simulink model "c09f12_01"  (R2012b)
settings: Solver=ode45  StartTime=0.0  StopTime="(2^(7+2))  * (2^8)"  RelTol=1e-3
undefined symbols (not defined in the file): Down, pfb_coeff_gen_calc, Up, xlipgetpartsetting
libraries: xbsIndex_r4 x7044, casper_library_misc x193, xps_library x58, casper_library_delays x50, simulink x16, dspsigops x12, casper_library_flow_control x5, xbsReplacements_r4 x4, casper_library_ffts_twiddle x2, casper_library_multipliers x2, casper_library_reorder x1
(part 6 of 77)

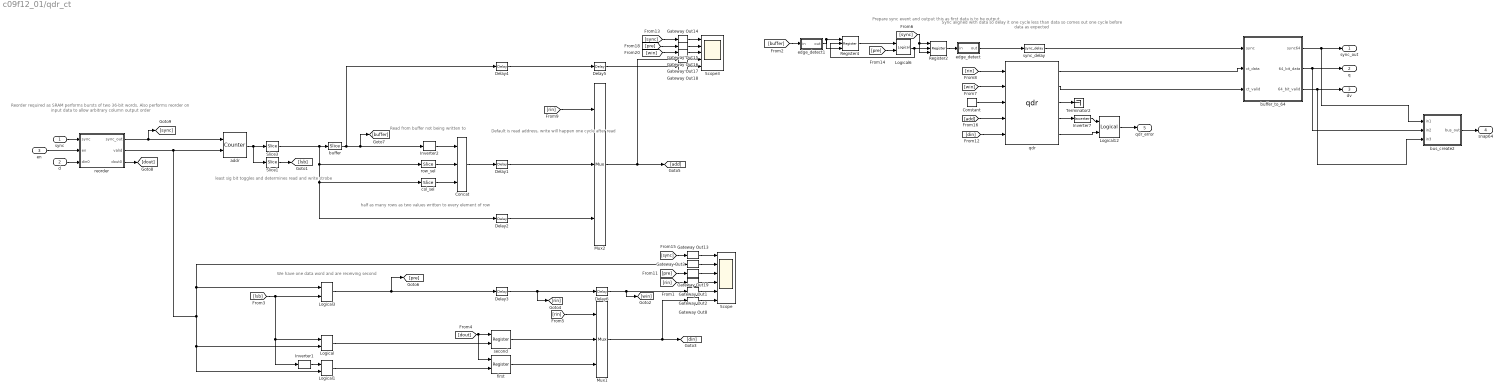
== system c09f12_01/qdr_ct ==
  note: Reorder required as SRAM performs
      | bursts of two 36-bit words.
      | Also performs reorder on input
      | data to allow arbitrary column
      | output order
  note: Prepare sync event and output
      | this as first data is to be output.
  note: Sync aligned with data so
      | delay it one cycle less
      | than data so comes out one
      | cycle before data as
      | expected
  note: least sig bit toggles
      | and determines read
      | and write strobe
  note: We have one data word
      | and are receiving second
  note: Default is read address,
      | write will happen one
      | cycle after read
  note: Read from buffer
      | not being
      | written to
  note: half as many rows
      | as two values
      | written to every
      | element of row
  sync : Inport
  d : Inport  Port=2
  en : Inport  Port=3
  Concat : xbsIndex_r4/Concat  num_inputs=3  dbl_ovrd=off  block_type=concat
      settings: block_version=10.1.3
  Constant : xbsIndex_r4/Constant  const=15  gui_display_data_type=Fixed-point  arith_type=Unsigned  n_bits=4  bin_pt=0  preci_type=Single  exp_width=8  frac_width=24  explicit_period=on  period=1  equ=P=C  opselect=C  inp2=PCIN>>17  opr=+  inp1=P  carry=CIN  dbl_ovrd=off  block_type=constant
  Delay{1..6} (6 alike) : xbsIndex_r4/Delay  rst=off  infoeditControl=Selection of Reset will increase slice count due to use of real FFs and instead of SRLs  en=off  latency=1  dbl_ovrd=off  reg_retiming=off  block_type=delay
      settings: block_version=11.4
  Gateway Out{1..3,8,13..19} (11 alike) : xbsIndex_r4/Gateway Out  inherit_from_input=off  hdl_port=off  timing_constraint=None  locs_specified=off  LOCs={}  UseAsDAC=off  DACChannel='1'  block_type=gatewayout
      settings: infoedit="Gateway out block.  Converts Xilinx fixed point inputs into ouputs of type Simulink integer, double, or fixed point.<br><br>Hardware notes:  In hardware these blocks become top level output ports or are discarded, depending on how they are configured."  block_version=11.4
  Inverter1 : xbsIndex_r4/Inverter  en=off  latency=0  dbl_ovrd=off  block_type=inv
  Inverter2 : xbsIndex_r4/Inverter  en=off  latency=0  dbl_ovrd=off  block_type=inv
  Inverter7 : xbsIndex_r4/Inverter  en=off  latency=0  dbl_ovrd=off  block_type=inv
      settings: block_version=11.4
  Logical{,1,3,6} (4 alike) : xbsIndex_r4/Logical  logical_function=AND  inputs=2  en=off  latency=0  precision=Full  arith_type=Unsigned  n_bits=16  bin_pt=0  align_bp=on  dbl_ovrd=off  block_type=logical
      settings: block_version=11.4
  Logical12 : xbsIndex_r4/Logical  logical_function=OR  inputs=2  en=off  latency=1  precision=Full  arith_type=Unsigned  n_bits=8  bin_pt=2  align_bp=on  dbl_ovrd=off  block_type=logical
      settings: xl_area=[0, 0, 0, 0, 0, 0, 0]
  Mux1 : xbsIndex_r4/Mux  inputs=2  en=off  latency=1  precision=Full  arith_type=Unsigned  n_bits=16  bin_pt=14  quantization=Truncate  overflow=Wrap  dbl_ovrd=off  block_type=mux
      settings: block_version=11.4
  Mux2 : xbsIndex_r4/Mux  inputs=2  en=off  latency=1  precision=Full  arith_type=Unsigned  n_bits=16  bin_pt=14  quantization=Truncate  overflow=Wrap  dbl_ovrd=off  block_type=mux
      settings: block_version=11.4
  Register2 : xbsIndex_r4/Register  init=0  rst=on  en=on  dbl_ovrd=off  block_type=register
      settings: block_version=11.4
  Register4 : xbsIndex_r4/Register  init=0  rst=on  en=on  dbl_ovrd=off  block_type=register
      settings: block_version=11.4
  Scope : Scope  NumInputPorts=6
      settings: YMin=0~0~0~0~0~0  YMax=1~1~1~1~1~15
  Scope3 : Scope  NumInputPorts=5
      settings: TimeRange=27.56125882301808  YMin=0~0~0~0~0  YMax=1~1~600~15~1  SaveName=ScopeData4
  Slice1 : xbsIndex_r4/Slice  nbits=1  boolean_output=on  mode=Lower Bit Location + Width  bit1=0  base1=MSB of Input  bit0=0  base0=LSB of Input  dbl_ovrd=off  block_type=slice
      settings: block_version=10.1.3
  Slice3 : xbsIndex_r4/Slice  nbits=(idepth + odepth + 1) - 1  boolean_output=off  mode=Upper Bit Location + Width  bit1=0  base1=MSB of Input  bit0=0  base0=LSB of Input  dbl_ovrd=off  block_type=slice
      settings: block_version=10.1.3
  Terminator2 : Terminator
  addr : xbsIndex_r4/Counter  cnt_type=Free Running  cnt_to=Inf  operation=Up  start_count=0  cnt_by_val=1  arith_type=Unsigned  n_bits=(idepth + odepth + 1)  bin_pt=0  load_pin=off  rst=on  en=on  explicit_period=on  period=1  dbl_ovrd=off  use_behavioral_HDL=off  implementation=Fabric  use_rpm=off  block_type=counter
  buffer : xbsIndex_r4/Slice  nbits=1  boolean_output=on  mode=Upper Bit Location + Width  bit1=0  base1=MSB of Input  bit0=0  base0=LSB of Input  dbl_ovrd=off  block_type=slice
      settings: block_version=10.1.3
  buffer_to_64 : Subsystem
  bus_create2 : Subsystem  AncestorBlock=casper_library_flow_control/bus_create  mask(bus_create){inputNum=3}
      mask prompts: inputNum "Number of inputs:"
      mask init:
      | bus_create_init(gcb,...
      |     'inputNum', inputNum);
  col_sel : xbsIndex_r4/Slice  nbits=idepth  boolean_output=off  mode=Lower Bit Location + Width  bit1=0  base1=MSB of Input  bit0=odepth-1  base0=LSB of Input  dbl_ovrd=off  block_type=slice
      settings: block_version=10.1.3
  edge_detect : Subsystem  AncestorBlock=casper_library_misc/edge_detect  mask(edge_detect){edge=Falling, polarity=Active High, x_in=[0 0.08 0.08 0.16 0.16 0.24 0.24 0.32 0.32 0.4], y_in=[1  1 -1 -1 -1 -1 -1 -1 -1 -1], x_out=[0.6 0.68 0.68 0.76 0.76 0.84 0.84 0.92 0.92 1], y_out=[-1 -1  1  1 -1 -1 -1 -1 -1 -1]}
      mask prompts: edge "Edge Type"; polarity "Output Polarity"; x_in "Input X Positions"; y_in "Input Y Positions"; x_out "Output X Positions"; y_out "Output Y Positions"
      mask help: Output is active for one-cycle after each edge of the specified type (i.e. rising, falling or both).
      mask init: same as c09f12_01/edge_detect2
      settings: AttributesFormatString=|
      | falling edges
      | active high
      mask Help: Output is active for one-cycle after each edge of the specified type (i.e. rising, falling, or both).  Latency is zero.
      mask TypeOptions edge: Rising | Falling | Both
      mask TypeOptions polarity: Active High | Active Low
      mask Display:
      | plot(x_in_num,0.5+y_in_num*0.2);
      | plot(x_out_num,0.5+y_out_num*0.2);
  edge_detect1 : Subsystem  AncestorBlock=casper_library_misc/edge_detect  mask(edge_detect){edge=Rising, polarity=Active High, x_in=[0 0.08 0.08 0.16 0.16 0.24 0.24 0.32 0.32 0.4], y_in=[-1 -1  1  1  1  1  1  1  1  1], x_out=[0.6 0.68 0.68 0.76 0.76 0.84 0.84 0.92 0.92 1], y_out=[-1 -1  1  1 -1 -1 -1 -1 -1 -1]}
      mask prompts: edge "Edge Type"; polarity "Output Polarity"; x_in "Input X Positions"; y_in "Input Y Positions"; x_out "Output X Positions"; y_out "Output Y Positions"
      mask help: Output is active for one-cycle after each edge of the specified type (i.e. rising, falling or both).
      mask init: same as c09f12_01/edge_detect2
      settings: AttributesFormatString=|
      | rising edges
      | active high
      mask Help: Output is active for one-cycle after each edge of the specified type (i.e. rising, falling, or both).  Latency is zero.
      mask TypeOptions edge: Rising | Falling | Both
      mask TypeOptions polarity: Active High | Active Low
      mask Display:
      | plot(x_in_num,0.5+y_in_num*0.2);
      | plot(x_out_num,0.5+y_out_num*0.2);
  first : xbsIndex_r4/Register  init=0  rst=off  en=on  dbl_ovrd=off  block_type=register
      settings: block_version=11.4
  qdr : xps_library/qdr  Tag=xps:qdr  which_qdr=qdr0  qdr_awidth=8  use_sniffer=off
  reorder : Subsystem  AncestorBlock=casper_library_reorder/reorder  mask(reorder){map=[2048  6144  2304  6400  2560  6656  2816  6912  3072  7168  3328  7424  3584  7680  3840  7936     0  4096   256  4352   512  4608   768  4864  1024  5120  1280  5376  1536  5632  1792  5888  2049  6145  2305  6401  2561  6657  2817  6913  3073  7169  3329  7425  3585  7681  3841  7937     1  4097   257  4353   513  4609   769  4865  1025  5121  1281  5377  1537  5633  1793  5889  2050  6146  2306  6402  2562  6658  2818  6914  3074  7170  3330  7426  3586  7682  3842  7938     2  4098   258  4354   514  4610   770  4866  1026  5122  1282  5378  1538  5634  1794  5890  2051  6147  2307  6403  2563  6659  2819  6915  3075  7171  3331  7427  3587  7683  3843  7939     3  4099   259  4355   515  4611   771  4867  1027  5123  1283  5379  1539  5635  1795  5891  2052  6148  2308  6404  2564  6660  2820  6916  3076  7172  3332  7428  3588  7684  3844  7940     4  4100   260  4356   516  4612   772  4868  1028  5124  1284  5380  1540  5636  1796  5892  2053  6149  2309  6405  2565  6661  2821  6917  3077  7173  3333  7429  3589  7685  3845  7941     5  4101   261  4357   517  4613   773  4869  1029  5125  1285  5381  1541  5637  1797  5893  2054  6150  2310  6406  2566  6662  2822  6918  3078  7174  3334  7430  3590  7686  3846  7942     6  4102   262  4358   518  4614   774  4870  1030  5126  1286  5382  1542  5638  1798  5894  2055  6151  2311  6407  2567  6663  2823  6919  3079  7175  3335  7431  3591  7687  3847  7943     7  4103   263  4359   519  4615   775  4871  1031  5127  1287  5383  1543  5639  1799  5895  2056  6152  2312  6408  2568  6664  2824  6920  3080  7176  3336  7432  3592  7688  3848  7944     8  4104   264  4360   520  4616   776  4872  1032  5128  1288  5384  1544  5640  1800  5896  2057  6153  2313  6409  2569  6665  2825  6921  3081  7177  3337  7433  3593  7689  3849  7945     9  4105   265  4361   521  4617   777  4873  1033  5129  1289  5385  1545  5641  1801  5897  2058  6154  2314  6410  2570  6666  2826  6922  3082  7178  3338  7434  3594  7690  3850  7946    10  4106   266  4362   522  4618   778  4874  1034  5130  1290  5386  1546  5642  1802  5898  2059  6155  2315  6411  2571  6667  2827  6923  3083  7179  3339  7435  3595  7691  3851  7947    11  4107   267  4363   523  4619   779  4875  1035  5131  1291  5387  1547  5643  1803  5899  2060  6156  2316  6412  2572  6668  2828  6924  3084  7180  3340  7436  3596  7692  3852  7948    12  4108   268  4364   524  4620   780  4876  1036  5132  1292  5388  1548  5644  1804  5900  2061  6157  2317  6413  2573  6669  2829  6925  3085  7181  3341  7437  3597  7693  3853  7949    13  4109   269  4365   525  4621   781  4877  1037  5133  1293  5389  1549  5645  1805  5901  2062  6158  2318  6414  2574  6670  2830  6926  3086  7182  3342  7438  3598  7694  3854  7950    14  4110   270  4366   526  4622   782  4878  1038  5134  1294  5390  1550  5646  1806  5902  2063  6159  2319  6415  2575  6671  2831  6927  3087  7183  3343  7439  3599  7695  3855  7951    15  4111   271  4367   527  4623   783  4879  1039  5135  1295  5391  1551  5647  1807  5903  2064  6160  2320  6416  2576  6672  2832  6928  3088  7184  3344  7440  3600  7696  3856  7952    16  4112   272  4368   528  4624   784  4880  1040  5136  1296  5392  1552  5648  1808  5904  2065  6161  2321  6417  2577  6673  2833  6929  3089  7185  3345  7441  3601  7697  3857  7953    17  4113   273  4369   529  4625   785  4881  1041  5137  1297  5393  1553  5649  1809  5905  2066  6162  2322  6418  2578  6674  2834  6930  3090  7186  3346  7442  3602  7698  3858  7954    18  4114   274  4370   530  4626   786  4882  1042  5138  1298  5394  1554  5650  1810  5906  2067  6163  2323  6419  2579  6675  2835  6931  3091  7187  3347  7443  3603  7699  3859  7955    19  4115   275  4371   531  4627   787  4883  1043  5139  1299  5395  1555  5651  1811  5907  2068  6164  2324  6420  2580  6676  2836  6932  3092  7188  3348  7444  3604  7700  3860  7956    20  4116   276  4372   532  4628   788  4884  1044  5140 ...(+45155 chars)], n_inputs=1, bram_latency=1, map_latency=1, double_buffer=1, bram_map=on}
      mask prompts: map "Output Order:"; n_inputs "Number of inputs"; bram_latency "BRAM Latency"; map_latency "Map Latency"; double_buffer "Double Buffer"; bram_map "Use BlockRAM for Map"
      mask init:
      | reorder_init(gcb, ...
      |     'map', map, ...
      |     'n_inputs', n_inputs, ...
      |     'bram_latency', bram_latency, ...
      |     'map_latency', map_latency, ...
      |     'double_buffer', double_buffer, ...
      |     'bram_map', bram_map);
      settings: AttributesFormatString=order=2
      mask Help: eval('xlWeb(''http://casper.berkeley.edu/wiki/Reorder'')')
  row_sel : xbsIndex_r4/Slice  nbits=odepth-1  boolean_output=off  mode=Lower Bit Location + Width  bit1=0  base1=MSB of Input  bit0=0  base0=LSB of Input  dbl_ovrd=off  block_type=slice
      settings: block_version=10.1.3
  second : xbsIndex_r4/Register  init=0  rst=off  en=on  dbl_ovrd=off  block_type=register
      settings: block_version=11.4
  sync_delay : casper_library_delays/sync_delay  DelayLen=10-1
  sync_out : Outport
  q : Outport  Port=2
  dv : Outport  Port=3
  snap64 : Outport  Port=4
  qdr_error : Outport  Port=5
  wires:
  sync/1 -> reorder/1(sync)
  en/1 -> reorder/2(en)
  [rin] -> qdr/1
  [win] -> qdr/2
  Constant/1 -> qdr/3
  [add] -> qdr/4
  qdr/5 -> Logical12/2
  qdr/4 -> Inverter7/1
  qdr/3 -> Terminator2/1
  qdr/2 -> buffer_to_64/3(ct_valid)
  sync_delay/1 -> buffer_to_64/1(sync)
  qdr/1 -> buffer_to_64/2(ct_data)
  addr/1 -> Slice1/1, Slice3/1
  Logical/1 -> second/2
  Logical1/1 -> first/2
  [rin] -> Mux1/1
  Mux1/1 -> [din], Gateway Out8/1
  [din] -> qdr/5
  buffer/1 -> [buffer], Inverter2/1, Delay4/1
  [sync] -> Register2/1, Register2/3
  Register4/1 -> Logical6/1
  [pre] -> Logical6/2
  Logical6/1 -> Register2/2, Register4/2
  Register2/1 -> edge_detect/1(in)
  edge_detect/1(out) -> sync_delay/1
  row_sel/1 -> Concat/2
  [rin] -> Mux2/1
  Concat/1 -> Delay1/1
  Inverter2/1 -> Concat/1
  [sync] -> Gateway Out13/1
  Delay3/1 -> [rin], Delay6/1
  [buffer] -> edge_detect1/1(in)
  edge_detect1/1(out) -> Register4/1, Register4/3
  col_sel/1 -> Concat/3
  second/1 -> Mux1/2
  first/1 -> Mux1/3
  Delay6/1 -> Gateway Out2/1, [win]
  [sync] -> Gateway Out14/1
  [pre] -> Gateway Out15/1
  [win] -> Gateway Out16/1
  Gateway Out14/1 -> Scope3/1
  Gateway Out15/1 -> Scope3/2
  Gateway Out16/1 -> Scope3/3
  Gateway Out17/1 -> Scope3/4
  Gateway Out18/1 -> Scope3/5
  Logical3/1 -> Delay3/1, [pre]
  [pre] -> Gateway Out19/1
  Gateway Out13/1 -> Scope/1
  Gateway Out3/1 -> Scope/2
  Gateway Out19/1 -> Scope/3
  Gateway Out1/1 -> Scope/4
  Gateway Out2/1 -> Scope/5
  Gateway Out8/1 -> Scope/6
  Inverter1/1 -> Logical1/1
  [rin] -> Gateway Out1/1
  Slice3/1 -> buffer/1, row_sel/1, col_sel/1, Delay2/1
  Slice1/1 -> [lsb]
  [lsb] -> Logical3/2, Inverter1/1, Logical/1
  Mux2/1 -> [add], Gateway Out17/1
  Delay1/1 -> Mux2/2
  Delay2/1 -> Mux2/3
  Delay4/1 -> Delay5/1
  Delay5/1 -> Gateway Out18/1
  reorder/2(valid) -> addr/2, Logical/2, Logical1/2, Gateway Out3/1, Logical3/1
  d/1 -> reorder/3(din0)
  reorder/3(dout0) -> [dout]
  [dout] -> second/1, first/1
  reorder/1(sync_out) -> [sync], addr/1
  buffer_to_64/1(sync64) -> sync_out/1, bus_create2/1(in1)
  buffer_to_64/2(64_bit_data) -> q/1, bus_create2/2(in2)
  buffer_to_64/3(64_bit_valid) -> dv/1, bus_create2/3(in3)
  bus_create2/1(bus_out) -> snap64/1
  Inverter7/1 -> Logical12/1
  Logical12/1 -> qdr_error/1
